simulink model "robot_2015_floor"  (R2017b)
(part 13 of 139)

  Revolute149/LConn1 -- upper_leg_casin_5_RIGID/RConn11
  Revolute149/RConn1 -- hex_bolt_gradeb_iso_274_RIGID/LConn1
  Revolute150/LConn1 -- upper_leg_casin_5_RIGID/RConn10
  Revolute150/RConn1 -- hex_bolt_gradeb_iso_275_RIGID/LConn1
  Revolute151/LConn1 -- upper_leg_casin_5_RIGID/RConn9
  Revolute23/RConn1 -- hex_nut_style_1_gradeab_iso_150_RIGID/LConn1
  Revolute151/RConn1 -- hex_bolt_gradeb_iso_276_RIGID/LConn1
  Revolute152/LConn1 -- upper_leg_casin_5_RIGID/RConn7
  Revolute152/RConn1 -- hex_bolt_gradeb_iso_277_RIGID/LConn1
  Revolute153/LConn1 -- upper_leg_casin_5_RIGID/RConn6
  Revolute153/RConn1 -- hex_bolt_gradeb_iso_278_RIGID/LConn1
  upper_leg_casin_6_RIGID/LConn1 -- upperleg_1_RIGID/LConn4
  Revolute154/LConn1 -- upper_leg_casin_6_RIGID/RConn10
  Revolute154/RConn1 -- hex_nut_style_1_gradeab_iso_261_RIGID/LConn1
  Revolute155/LConn1 -- upper_leg_casin_6_RIGID/RConn9
  Revolute155/RConn1 -- hex_nut_style_1_gradeab_iso_262_RIGID/LConn1
  Lower_joint_cap_1_RIGID/RConn2 -- Revolute24/LConn1
  Revolute156/LConn1 -- upper_leg_casin_6_RIGID/RConn7
  Revolute156/RConn1 -- hex_nut_style_1_gradeab_iso_263_RIGID/LConn1
  Revolute157/LConn1 -- upper_leg_casin_6_RIGID/RConn6
  Revolute157/RConn1 -- hex_nut_style_1_gradeab_iso_264_RIGID/LConn1
  Revolute158/LConn1 -- upper_leg_casin_6_RIGID/RConn5
  Revolute158/RConn1 -- hex_nut_style_1_gradeab_iso_265_RIGID/LConn1
  Revolute159/LConn1 -- upper_leg_casin_6_RIGID/RConn4
  Revolute159/RConn1 -- hex_nut_style_1_gradeab_iso_266_RIGID/LConn1
  Revolute160/LConn1 -- upper_leg_casin_6_RIGID/RConn1
  Revolute160/RConn1 -- hex_bolt_gradeb_iso_267_RIGID/LConn1
  Revolute24/RConn1 -- hex_nut_style_1_gradeab_iso_159_RIGID/LConn1
  Revolute161/LConn1 -- upper_leg_casin_6_RIGID/RConn13
  Revolute161/RConn1 -- hex_bolt_gradeb_iso_268_RIGID/LConn1
  Revolute162/LConn1 -- upper_leg_casin_6_RIGID/RConn12
  Revolute162/RConn1 -- hex_bolt_gradeb_iso_269_RIGID/LConn1
  Revolute163/LConn1 -- upper_leg_casin_6_RIGID/RConn2
  Revolute163/RConn1 -- hex_bolt_gradeb_iso_270_RIGID/LConn1
  Revolute164/LConn1 -- upper_leg_casin_6_RIGID/RConn11
  Revolute164/RConn1 -- hex_bolt_gradeb_iso_271_RIGID/LConn1
  Revolute165/LConn1 -- upper_leg_casin_6_RIGID/RConn3
  Revolute165/RConn1 -- hex_bolt_gradeb_iso_272_RIGID/LConn1
  Lower_joint_cap_1_RIGID/RConn1 -- Revolute25/LConn1
  Revolute166/LConn1 -- upper_leg_casin_7_RIGID/RConn6
  Revolute166/RConn1 -- hex_bolt_gradeb_iso_249_RIGID/LConn1
  Revolute167/LConn1 -- upper_leg_casin_7_RIGID/RConn5
  Revolute167/RConn1 -- hex_bolt_gradeb_iso_250_RIGID/LConn1
  Revolute168/LConn1 -- upper_leg_casin_7_RIGID/RConn4
  Revolute168/RConn1 -- hex_bolt_gradeb_iso_251_RIGID/LConn1
  Revolute169/LConn1 -- upper_leg_casin_7_RIGID/RConn3
  Revolute169/RConn1 -- hex_bolt_gradeb_iso_252_RIGID/LConn1
  Revolute170/LConn1 -- upper_leg_casin_7_RIGID/RConn1
  Revolute170/RConn1 -- hex_bolt_gradeb_iso_253_RIGID/LConn1
  Revolute25/RConn1 -- hex_nut_style_1_gradeab_iso_160_RIGID/LConn1
  Revolute171/LConn1 -- upper_leg_casin_7_RIGID/RConn2
  Revolute171/RConn1 -- hex_bolt_gradeb_iso_254_RIGID/LConn1
  Prismatic7/LConn1 -- upper_leg_cap_1_RIGID/RConn2
  Prismatic7/RConn1 -- upper_leg_casin_7_RIGID/LConn2
  Prismatic8/LConn1 -- motor_axle_1_RIGID/RConn1
  Prismatic8/RConn1 -- SEA_system_hip_1_RIGID/LConn2
  Rectangular2/LConn1 -- hip_1_RIGID/RConn25
  Rectangular2/RConn1 -- SEA_system_hip_1_RIGID/LConn1
  Lower_joint_casin_1_RIGID/RConn12 -- Prismatic9/LConn1
  Prismatic9/RConn1 -- beam_filler_1_RIGID/LConn1
  Ball_bearing_filler_2_RIGID/LConn1 -- Lower_joint_cap_1_RIGID/LConn1
  beam_filler_1_RIGID/LConn2 -- upperleg_1_RIGID/LConn3
  Lower_joint_casin_2_RIGID/LConn2 -- beam_filler_2_RIGID/LConn1
  beam_filler_2_RIGID/LConn2 -- upperleg_1_RIGID/LConn1
  Lower_joint_casin_5_RIGID/LConn3 -- beam_filler_3_RIGID/LConn1
  beam_filler_3_RIGID/LConn2 -- lower_leg_main_1_RIGID/LConn1
  Revolute172/LConn1 -- beam_filler_4_RIGID/RConn2
  Lower_joint_casin_3_RIGID/LConn2 -- Revolute172/RConn1
  Prismatic10/LConn1 -- beam_filler_4_RIGID/RConn1
  Prismatic10/RConn1 -- lower_leg_main_1_RIGID/LConn3
  Planar56/LConn1 -- upper_leg_cap_1_RIGID/RConn1
  Lower_joint_cap_2_RIGID/RConn6 -- Planar6/LConn1
  Planar56/RConn1 -- bearing_1_RIGID/LConn1
  Ball_bearing_filler_small_1_RIGID/LConn2 -- upper_leg_cap_1_RIGID/LConn1
  Planar57/LConn1 -- upper_leg_cap_2_RIGID/RConn6
  Planar57/RConn1 -- hex_nut_style_1_gradeab_iso_164_RIGID/LConn1
  Planar58/LConn1 -- upper_leg_cap_2_RIGID/RConn5
  Planar58/RConn1 -- hex_nut_style_1_gradeab_iso_165_RIGID/LConn1
  Planar59/LConn1 -- upper_leg_cap_2_RIGID/RConn2
  Planar59/RConn1 -- hex_nut_style_1_gradeab_iso_166_RIGID/LConn2
  Planar60/LConn1 -- upper_leg_cap_2_RIGID/RConn1
  Planar60/RConn1 -- hex_nut_style_1_gradeab_iso_168_RIGID/LConn2
  Planar6/RConn1 -- hex_nut_style_1_gradeab_iso_161_RIGID/LConn1
  Planar61/LConn1 -- upper_leg_cap_2_RIGID/RConn4
  Planar61/RConn1 -- hex_nut_style_1_gradeab_iso_169_RIGID/LConn1
  Planar62/LConn1 -- upper_leg_cap_2_RIGID/RConn3
  Planar62/RConn1 -- hex_nut_style_1_gradeab_iso_170_RIGID/LConn1
  Ball_bearing_filler_small_1_RIGID/LConn1 -- upper_leg_cap_2_RIGID/LConn1
  Revolute173/LConn1 -- bearing_3_RIGID/RConn1
  Revolute173/RConn1 -- upper_leg_cap_3_RIGID/LConn2
  Ball_bearing_filler_small_4_RIGID/LConn2 -- upper_leg_cap_3_RIGID/LConn1
  Revolute174/LConn1 -- upper_leg_cap_4_RIGID/RConn2
  Revolute174/RConn1 -- bearing_4_RIGID/LConn1
  Lower_joint_cap_2_RIGID/RConn3 -- Planar7/LConn1
  Ball_bearing_filler_small_3_RIGID/LConn2 -- upper_leg_cap_4_RIGID/LConn1
  Revolute175/LConn1 -- upper_leg_cap_5_RIGID/RConn6
  Revolute175/RConn1 -- hex_nut_style_1_gradeab_iso_198_RIGID/LConn1
  Revolute176/LConn1 -- upper_leg_cap_5_RIGID/RConn5
  Revolute176/RConn1 -- hex_nut_style_1_gradeab_iso_200_RIGID/LConn1
  Revolute177/LConn1 -- upper_leg_cap_5_RIGID/RConn4
  Revolute177/RConn1 -- hex_nut_style_1_gradeab_iso_202_RIGID/LConn1
  Revolute178/LConn1 -- upper_leg_cap_5_RIGID/RConn3
  Revolute178/RConn1 -- hex_nut_style_1_gradeab_iso_203_RIGID/LConn1
  Revolute179/LConn1 -- upper_leg_cap_5_RIGID/RConn2
  Revolute3/LConn1 -- hip_joint_casin_1_RIGID/RConn6
  Planar7/RConn1 -- hex_nut_style_1_gradeab_iso_162_RIGID/LConn2
  Revolute179/RConn1 -- hex_nut_style_1_gradeab_iso_207_RIGID/LConn1
  Revolute180/LConn1 -- upper_leg_cap_5_RIGID/RConn1
  Revolute180/RConn1 -- hex_nut_style_1_gradeab_iso_208_RIGID/LConn1
  Ball_bearing_filler_small_6_RIGID/LConn1 -- upper_leg_cap_5_RIGID/LConn1
  Planar63/LConn1 -- upper_leg_cap_6_RIGID/RConn6
  Planar63/RConn1 -- hex_nut_style_1_gradeab_iso_215_RIGID/LConn1
  Planar64/LConn1 -- upper_leg_cap_6_RIGID/RConn3
  Planar64/RConn1 -- hex_nut_style_1_gradeab_iso_216_RIGID/LConn2
  Planar65/LConn1 -- upper_leg_cap_6_RIGID/RConn5
  Planar65/RConn1 -- hex_nut_style_1_gradeab_iso_217_RIGID/LConn1
  Lower_joint_cap_2_RIGID/RConn5 -- Planar8/LConn1
  Planar66/LConn1 -- upper_leg_cap_6_RIGID/RConn2
  Planar66/RConn1 -- hex_nut_style_1_gradeab_iso_218_RIGID/LConn2
  Planar67/LConn1 -- upper_leg_cap_6_RIGID/RConn1
  Planar67/RConn1 -- hex_nut_style_1_gradeab_iso_219_RIGID/LConn2
  Planar68/LConn1 -- upper_leg_cap_6_RIGID/RConn4
  Planar68/RConn1 -- hex_nut_style_1_gradeab_iso_220_RIGID/LConn1
  Ball_bearing_filler_small_5_RIGID/LConn2 -- upper_leg_cap_6_RIGID/LConn1
  Planar69/LConn1 -- bearing_2_RIGID/RConn2
  Planar69/RConn1 -- upper_leg_cap_7_RIGID/LConn1
  Ball_bearing_filler_small_2_RIGID/LConn1 -- upper_leg_cap_7_RIGID/LConn3
  Planar8/RConn1 -- hex_nut_style_1_gradeab_iso_163_RIGID/LConn1
  Planar70/LConn1 -- upper_leg_cap_8_RIGID/RConn6
  Planar70/RConn1 -- hex_nut_style_1_gradeab_iso_151_RIGID/LConn1
  Planar71/LConn1 -- upper_leg_cap_8_RIGID/RConn5
  Planar71/RConn1 -- hex_nut_style_1_gradeab_iso_152_RIGID/LConn1
  Planar72/LConn1 -- upper_leg_cap_8_RIGID/RConn4
  Planar72/RConn1 -- hex_nut_style_1_gradeab_iso_153_RIGID/LConn1
  Planar73/LConn1 -- upper_leg_cap_8_RIGID/RConn2
  Planar73/RConn1 -- hex_nut_style_1_gradeab_iso_154_RIGID/LConn2
  Planar74/LConn1 -- upper_leg_cap_8_RIGID/RConn3
  Planar74/RConn1 -- hex_nut_style_1_gradeab_iso_156_RIGID/LConn1
  Lower_joint_cap_2_RIGID/RConn4 -- Planar9/LConn1
  Planar75/LConn1 -- upper_leg_cap_8_RIGID/RConn1
  Planar75/RConn1 -- hex_nut_style_1_gradeab_iso_158_RIGID/LConn1
  Ball_bearing_filler_small_2_RIGID/LConn3 -- upper_leg_cap_8_RIGID/LConn1
  Planar76/LConn1 -- upper_leg_cap_9_RIGID/RConn6
  Planar76/RConn1 -- hex_nut_style_1_gradeab_iso_191_RIGID/LConn1
  Planar77/LConn1 -- upper_leg_cap_9_RIGID/RConn4
  Planar77/RConn1 -- hex_nut_style_1_gradeab_iso_192_RIGID/LConn1
  Planar78/LConn1 -- upper_leg_cap_9_RIGID/RConn5
  Planar78/RConn1 -- hex_nut_style_1_gradeab_iso_193_RIGID/LConn1
  Planar79/LConn1 -- upper_leg_cap_9_RIGID/RConn3
  Planar9/RConn1 -- hex_nut_style_1_gradeab_iso_167_RIGID/LConn1
  Planar79/RConn1 -- hex_nut_style_1_gradeab_iso_194_RIGID/LConn1
  Planar80/LConn1 -- upper_leg_cap_9_RIGID/RConn2
  Planar80/RConn1 -- hex_nut_style_1_gradeab_iso_195_RIGID/LConn2
  Planar81/LConn1 -- upper_leg_cap_9_RIGID/RConn1
  Planar81/RConn1 -- hex_nut_style_1_gradeab_iso_196_RIGID/LConn2
  Ball_bearing_filler_small_3_RIGID/LConn1 -- upper_leg_cap_9_RIGID/LConn1
  Revolute181/LConn1 -- hip_joint_casin_2_RIGID/RConn4
  Ball_bearing_filler_1_RIGID/LConn2 -- Revolute181/RConn1
  Cylindrical79/LConn1 -- bearing_1_RIGID/RConn2
  Ball_bearing_filler_1_RIGID/LConn1 -- Cylindrical79/RConn1
  Lower_joint_cap_2_RIGID/RConn2 -- Planar10/LConn1
  Revolute182/LConn1 -- hip_joint_casin_1_RIGID/RConn9
  Ball_bearing_filler_2_RIGID/LConn2 -- Revolute182/RConn1
  Cylindrical80/LConn1 -- bearing_2_RIGID/RConn1
  Ball_bearing_filler_2_RIGID/LConn3 -- Cylindrical80/RConn1
  Ball_bearing_filler_3_RIGID/LConn2 -- Lower_joint_casin_2_RIGID/LConn1
  Ball_bearing_filler_4_RIGID/LConn2 -- Lower_joint_casin_1_RIGID/LConn1
  Ball_bearing_filler_5_RIGID/LConn1 -- Lower_joint_casin_3_RIGID/LConn1
  Ball_bearing_filler_6_RIGID/RConn1 -- Revolute183/LConn1
  Lower_joint_casin_5_RIGID/LConn1 -- Revolute183/RConn1
  Cylindrical81/LConn1 -- bearing_6_RIGID/RConn1
  Planar10/RConn1 -- hex_nut_style_1_gradeab_iso_171_RIGID/LConn2
  Ball_bearing_filler_6_RIGID/LConn1 -- Cylindrical81/RConn1
  beam_filler_hip_1_RIGID/LConn1 -- hip_1_RIGID/LConn4
  beam_filler_hip_2_RIGID/LConn2 -- hip_1_RIGID/LConn1
  Revolute184/LConn1 -- hip_1_RIGID/RConn6
  Revolute184/RConn1 -- hex_bolt_gradeb_iso_145_RIGID/LConn1
  Revolute185/LConn1 -- hip_1_RIGID/RConn5
  Revolute185/RConn1 -- hex_bolt_gradeb_iso_146_RIGID/LConn1
  Revolute186/LConn1 -- hip_1_RIGID/RConn7
  Revolute186/RConn1 -- hex_bolt_gradeb_iso_147_RIGID/LConn1
  Revolute187/LConn1 -- hip_1_RIGID/RConn4
  Lower_joint_cap_2_RIGID/RConn1 -- Planar11/LConn1
  Revolute187/RConn1 -- hex_bolt_gradeb_iso_148_RIGID/LConn1
  Revolute188/LConn1 -- hip_1_RIGID/RConn2
  Revolute188/RConn1 -- hex_bolt_gradeb_iso_149_RIGID/LConn1
  Revolute189/LConn1 -- hip_1_RIGID/RConn3
  Revolute189/RConn1 -- hex_bolt_gradeb_iso_150_RIGID/LConn1
  Revolute190/LConn1 -- hip_1_RIGID/RConn1
  Revolute190/RConn1 -- hex_bolt_gradeb_iso_151_RIGID/LConn1
  Revolute191/LConn1 -- hip_1_RIGID/RConn24
  Revolute191/RConn1 -- hex_bolt_gradeb_iso_152_RIGID/LConn1
  Revolute192/LConn1 -- hip_1_RIGID/RConn23
  Planar11/RConn1 -- hex_nut_style_1_gradeab_iso_172_RIGID/LConn2
  Revolute192/RConn1 -- hex_bolt_gradeb_iso_153_RIGID/LConn1
  Revolute193/LConn1 -- hip_1_RIGID/RConn22
  Revolute193/RConn1 -- hex_bolt_gradeb_iso_154_RIGID/LConn1
  Revolute194/LConn1 -- hip_1_RIGID/RConn21
  Revolute194/RConn1 -- hex_bolt_gradeb_iso_155_RIGID/LConn1
  Revolute195/LConn1 -- hip_1_RIGID/RConn20
  Revolute195/RConn1 -- hex_bolt_gradeb_iso_156_RIGID/LConn1
  Revolute196/LConn1 -- hip_1_RIGID/RConn19
  Revolute196/RConn1 -- hex_bolt_gradeb_iso_157_RIGID/LConn1
  Revolute197/LConn1 -- hip_1_RIGID/RConn18
  Ball_bearing_filler_1_RIGID/LConn3 -- Lower_joint_cap_2_RIGID/LConn1
  Revolute197/RConn1 -- hex_bolt_gradeb_iso_158_RIGID/LConn1
  Revolute198/LConn1 -- hip_1_RIGID/RConn16
  Revolute198/RConn1 -- hex_bolt_gradeb_iso_159_RIGID/LConn1
  Revolute199/LConn1 -- hip_1_RIGID/RConn17
  Revolute199/RConn1 -- hex_bolt_gradeb_iso_160_RIGID/LConn1
  Revolute200/LConn1 -- hip_1_RIGID/RConn15
  Revolute200/RConn1 -- hex_bolt_gradeb_iso_161_RIGID/LConn1
  Revolute201/LConn1 -- hip_1_RIGID/RConn14
  Revolute201/RConn1 -- hex_bolt_gradeb_iso_162_RIGID/LConn1
  Revolute202/LConn1 -- hip_1_RIGID/RConn13
  Revolute3/RConn1 -- hex_nut_style_1_gradeab_iso_251_RIGID/LConn1
  Lower_joint_cap_3_RIGID/RConn6 -- Revolute26/LConn1
  Revolute202/RConn1 -- hex_bolt_gradeb_iso_163_RIGID/LConn1
  Revolute203/LConn1 -- hip_1_RIGID/RConn12
  Revolute203/RConn1 -- hex_bolt_gradeb_iso_164_RIGID/LConn1
  Revolute204/LConn1 -- hip_1_RIGID/RConn11
  Revolute204/RConn1 -- hex_bolt_gradeb_iso_165_RIGID/LConn1
  Revolute205/LConn1 -- hip_1_RIGID/RConn10
  Revolute205/RConn1 -- hex_bolt_gradeb_iso_166_RIGID/LConn1
  Revolute206/LConn1 -- hip_1_RIGID/RConn9
  Revolute206/RConn1 -- hex_bolt_gradeb_iso_167_RIGID/LConn1
  Revolute207/LConn1 -- hip_1_RIGID/RConn8
  Revolute26/RConn1 -- hex_nut_style_1_gradeab_iso_173_RIGID/LConn1
  Revolute207/RConn1 -- hex_bolt_gradeb_iso_168_RIGID/LConn1
  hip_1_RIGID/LConn3 -- upper_leg_casin_3_RIGID/LConn1
  hip_1_RIGID/LConn2 -- upper_leg_casin_4_RIGID/LConn1
  upper_leg_casin_2_RIGID/LConn4 -- F/RConn1
  upper_leg_casin_7_RIGID/LConn1 -- F1/RConn1
  Lower_joint_cap_3_RIGID/RConn5 -- Revolute27/LConn1
  Revolute27/RConn1 -- hex_nut_style_1_gradeab_iso_174_RIGID/LConn1
  Lower_joint_cap_3_RIGID/RConn4 -- Revolute28/LConn1
  Revolute28/RConn1 -- hex_nut_style_1_gradeab_iso_177_RIGID/LConn1
  Lower_joint_cap_3_RIGID/RConn3 -- Revolute29/LConn1
  Revolute29/RConn1 -- hex_nut_style_1_gradeab_iso_180_RIGID/LConn1
  Lower_joint_cap_3_RIGID/RConn2 -- Revolute30/LConn1
  Revolute30/RConn1 -- hex_nut_style_1_gradeab_iso_181_RIGID/LConn1
  Revolute4/LConn1 -- hip_joint_casin_1_RIGID/RConn5
  Lower_joint_cap_3_RIGID/RConn1 -- Revolute31/LConn1
  Revolute31/RConn1 -- hex_nut_style_1_gradeab_iso_184_RIGID/LConn1
  Ball_bearing_filler_4_RIGID/LConn1 -- Lower_joint_cap_3_RIGID/LConn1
  Lower_joint_cap_4_RIGID/RConn4 -- Planar12/LConn1
  Planar12/RConn1 -- hex_nut_style_1_gradeab_iso_185_RIGID/LConn2
  Lower_joint_cap_4_RIGID/RConn6 -- Planar13/LConn1
  Planar13/RConn1 -- hex_nut_style_1_gradeab_iso_186_RIGID/LConn1
  Lower_joint_cap_4_RIGID/RConn5 -- Planar14/LConn1
  Planar14/RConn1 -- hex_nut_style_1_gradeab_iso_187_RIGID/LConn1
  Lower_joint_cap_4_RIGID/RConn3 -- Planar15/LConn1
  "rightLegController "/RConn1 -- Revolute44/LConn2
  "rightLegController "/RConn2 -- Revolute45/LConn2
  "rightLegController "/RConn3 -- Revolute46/LConn2
  Revolute44/RConn2 -- "rightLegController "/LConn1
  Revolute44/RConn3 -- "rightLegController "/LConn2
  Revolute45/RConn2 -- "rightLegController "/LConn3
  Revolute45/RConn3 -- "rightLegController "/LConn4
  Revolute46/RConn2 -- "rightLegController "/LConn5
  Revolute46/RConn3 -- "rightLegController "/LConn6
